simulink subsystem "PvtSubSys_PLAN_ALC"  (R2020b)
settings: Solver=VariableStepAuto  StartTime=0.0  StopTime=10.0  RelTol=1e-3
undefined symbols (not defined in the file or in its folder): P_Global_WheelBase_m, P_Global_WheelTrack_m, P_PLAN_ALC_DPCConfirmTimeHMI, P_PLAN_ALC_DPCExtraMultiFrameConfirmCntDrv, P_PLAN_ALC_DPCExtraMultiFrameConfirmCntNoh, P_PLAN_ALC_DPCExtraMultiFrameConfirmCntOverTk, P_PLAN_ALC_DPCthresholdLcDrvLv1, P_PLAN_ALC_DPCthresholdLcDrvLv2, P_PLAN_ALC_DPCthresholdLcDrvLv3, P_PLAN_ALC_DynamicDPCthreshold, P_PLAN_ALC_FWheelPreTime, P_PLAN_ALC_LcCancelDPCThreshold, P_PLAN_ALC_LcCancelLaneChangeReqDspTimeCnt, P_PLAN_ALC_LcCancelRoadWidthOffset, P_PLAN_ALC_LcCancelRoadWidthOffsetForDPC, P_PLAN_ALC_LcCurvatureInhibitionValueBrkPoints, P_PLAN_ALC_LcCurvatureInhibitionValueTable, P_PLAN_ALC_LcDelayCntSetNoh, P_PLAN_ALC_LcDelayCntSetOverTk, P_PLAN_ALC_LCDeltaTmeGap, P_PLAN_ALC_LcDrv_DyDiffThreshold, P_PLAN_ALC_LcDrvHMILineValidFtime, P_PLAN_ALC_LcEnterLane_factor, P_PLAN_ALC_LcFinishDyDiffBrkPoint, P_PLAN_ALC_LcFinishDyDiffRwFactorForAP, P_PLAN_ALC_LcFinishDyDiffRwFactorForHMI, P_PLAN_ALC_LcFinishDyDiffTableValue, P_PLAN_ALC_LciDrvExistDefaultDisp, P_PLAN_ALC_LciOverTkDeltaSpdLv1, P_PLAN_ALC_LciOverTkDeltaSpdLv2, P_PLAN_ALC_LciOverTkDeltaSpdLv3, P_PLAN_ALC_LcOverTkDPCthreshold, P_PLAN_ALC_LcOverTkRearVehTTClimit, P_PLAN_ALC_NOHLcSwt, P_PLAN_ALC_NOHTurnSts, P_PLAN_ALC_OverTkCutOutDyRWFactor, P_PLAN_ALC_OveTkrSupDist, P_PLAN_ALC_PreCurvatureFactor, P_PLAN_ALC_PreCurvaturePreTime, P_PLAN_ALC_TurnLmpType, P_PLAN_ALC_vMinPreLC_Drv, P_PLAN_ALC_vMinPreLC_Noh, P_PLAN_ALC_vMinPreLC_OverTk, P_PLAN_LcCancelTestEnable, PLAN_ALC_DangerObjIndex, PLAN_ALC_LcCancelReason, PLAN_ALC_LcDecsLe, PLAN_ALC_LcDecsRi, PLAN_ALC_LcFeReason, PLAN_ALC_LcReason, PLAN_ALC_sts, PLAN_ALC_stsReason, PLAN_ALC_TurnLightReq
libraries: simulink x198, TrueDurationTime x21, RisingEdgeTimer x2, JumpDetectionUint x1
(part 3 of 4)

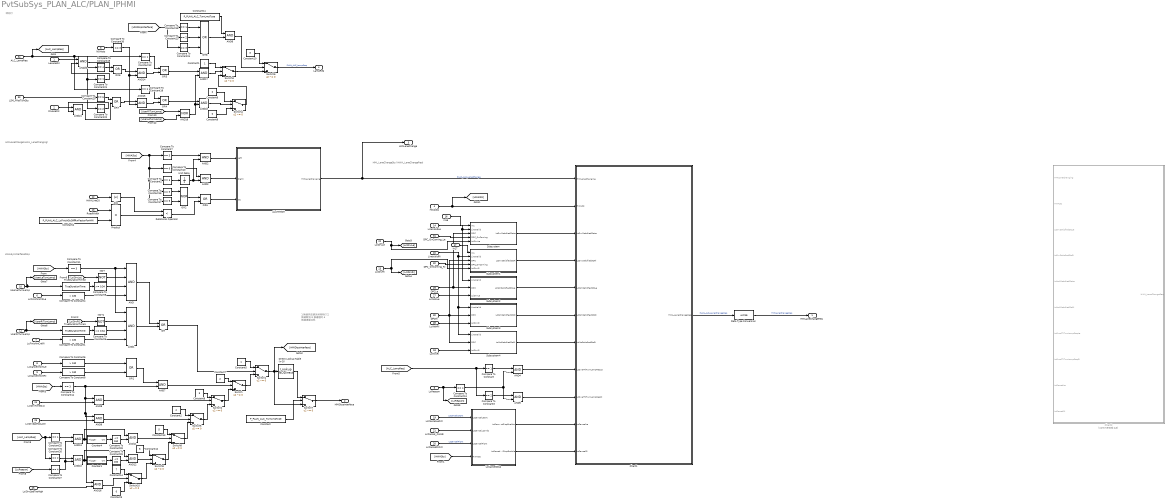
== system PvtSubSys_PLAN_ALC/PLAN_IPHMI ==
  note: 1 换道完成请关闭转向灯
      | 2 换道取消
      | 3 换道超时
      | 4 换道速度过低
  note: 转向灯
  note: HMILaneChange(HWA_LaneChanging)
  note: HMI_LaneChangeSts (HWA_LaneChangeReq)
  note: HWASysInterfaceDisp
  LeLaneOK : Inport
  RiLaneOK : Inport  Port=2
  NOHsts : Inport  Port=3
  HWASts : Inport  Port=4
  LcReason : Inport  Port=5
  LcFinishInCntLe : Inport  Port=6
  LcFinishInCntRi : Inport  Port=7
  LcCancelInCntLe : Inport  Port=8
  LcCancelInCntRi : Inport  Port=9
  UserLeTurnLamp : Inport  Port=10
  UserRiTurnLamp : Inport  Port=11
  HWALineC0 : Inport  Port=12
  RoadWidth : Inport  Port=13
  LineValidLe : Inport  Port=14
  LineValidRi : Inport  Port=15
  In16 : Inport  Port=16
  In17 : Inport  Port=17
  LcMrcRi : Inport  Port=18
  LcCancelLeCnt : Inport  Port=19
  LcCancelRiCnt : Inport  Port=20
  LcCancel_Conds : Inport  Port=21
  LciDrvLe : Inport  Port=22
  LciDrvRi : Inport  Port=23
  LciDrvTimeOut : Inport  Port=24
  LciDrvSpdTooLoW : Inport  Port=25
  LciDrvSpdTooHigh : Inport  Port=26
  LciNohLe : Inport  Port=27
  LciNohRi : Inport  Port=28
  DPCLe : Inport  Port=29
  DPCRi : Inport  Port=30
  DPC_OnComing_Le : Inport  Port=31
  DPC_OnComing_Ri : Inport  Port=32
  LSM_PilotTurnSts : Inport  Port=33
  ALC_LampReq : Inport  Port=34
  ALCHMISM : Stateflow chart  TreatAsAtomicUnit=on
  AND : Logic  Inputs=4  AllPortsSameDT=off  OutDataTypeStr=boolean
  AND1 : Logic  Inputs=4  AllPortsSameDT=off  OutDataTypeStr=boolean
  AND{2..3,6..18,20..21} (17 alike) : Logic  AllPortsSameDT=off  OutDataTypeStr=boolean
  AND19 : Logic  Operator=NOR  AllPortsSameDT=off  OutDataTypeStr=boolean
  AND4 : Logic  IconShape=distinctive  AllPortsSameDT=off  OutDataTypeStr=boolean
  AND5 : Logic  IconShape=distinctive  AllPortsSameDT=off  OutDataTypeStr=boolean
  Abs : Abs
  Chart1 : Stateflow chart  TreatAsAtomicUnit=on
  Chart2 : Stateflow chart  Commented=on  TreatAsAtomicUnit=on
  Compare To Constant{,12,15,21,25} (5 alike) : simulink/Logic and Bit Operations/Compare To Constant  relop===  const=1  OutDataTypeStr=boolean
  Compare To Constant{1,4,6,8} (4 alike) : simulink/Logic and Bit Operations/Compare To Constant  relop=>  const=130  OutDataTypeStr=boolean
  Compare To Constant10 : simulink/Logic and Bit Operations/Compare To Constant  relop===  const=6  OutDataTypeStr=boolean
  Compare To Constant{2,11,14,24,30} (5 alike) : simulink/Logic and Bit Operations/Compare To Constant  relop===  const=3  OutDataTypeStr=boolean
  Compare To Constant13 : simulink/Logic and Bit Operations/Compare To Constant  relop===  const=4  OutDataTypeStr=boolean
  Compare To Constant16 : simulink/Logic and Bit Operations/Compare To Constant  relop===  const=5  OutDataTypeStr=boolean
  Compare To Constant17 : simulink/Logic and Bit Operations/Compare To Constant  relop===  const=6  OutDataTypeStr=boolean
  Compare To Constant{3,18,22..23,26} (5 alike) : simulink/Logic and Bit Operations/Compare To Constant  relop===  const=2  OutDataTypeStr=boolean
  Compare To Constant19 : simulink/Logic and Bit Operations/Compare To Constant  relop===  const=4  OutDataTypeStr=boolean
  Compare To Constant20 : simulink/Logic and Bit Operations/Compare To Constant  relop===  const=5  OutDataTypeStr=boolean
  Compare To Constant27 : simulink/Logic and Bit Operations/Compare To Constant  relop===  const=4  OutDataTypeStr=boolean
  Compare To Constant28 : simulink/Logic and Bit Operations/Compare To Constant  relop=<=  const=150  OutDataTypeStr=boolean
  Compare To Constant29 : simulink/Logic and Bit Operations/Compare To Constant  relop=<=  const=150  OutDataTypeStr=boolean
  Compare To Constant5 : simulink/Logic and Bit Operations/Compare To Constant  relop=>=  const=0.34  OutDataTypeStr=boolean
  Compare To Constant7 : simulink/Logic and Bit Operations/Compare To Constant  relop===  const=5  OutDataTypeStr=boolean
  Compare To Constant9 : simulink/Logic and Bit Operations/Compare To Constant  relop=>=  const=0.34  OutDataTypeStr=boolean
  Constant : Constant  Value=P_PLAN_ALC_TurnLmpType
  Constant1 : Constant  OutDataTypeStr=uint8
  Constant10 : Constant  Value=3  OutDataTypeStr=uint8
  Constant11 : Constant  Value=P_PLAN_ALC_TurnLmpType
  Constant12 : Constant  Value=6  OutDataTypeStr=Inherit: Inherit via back propagation
  Constant13 : Constant  Value=5  OutDataTypeStr=Inherit: Inherit via back propagation
  Constant14 : Constant  Value=7  OutDataTypeStr=Inherit: Inherit via back propagation
  Constant2 : Constant  Value=4  OutDataTypeStr=Inherit: Inherit via back propagation
  Constant3 : Constant  Value=0  OutDataTypeStr=Inherit: Inherit via back propagation
  Constant4 : Constant  Value=P_PLAN_ALC_LcFinishDyDiffRwFactorForHMI
  Constant5 : Constant  OutDataTypeStr=Inherit: Inherit via back propagation
  Constant6 : Constant  Value=2  OutDataTypeStr=uint8
  Constant7 : Constant  Value=2  OutDataTypeStr=Inherit: Inherit via back propagation
  Constant8 : Constant  Value=3  OutDataTypeStr=Inherit: Inherit via back propagation
  Constant9 : Constant  Value=0  OutDataTypeStr=uint8
  Counter1 : Subsystem
  Counter4 : Subsystem
  Data Type Conversion : DataTypeConversion  OutDataTypeStr=uint16
  Direct Lookup Table (n-D) : LookupNDDirect  NumberOfTableDimensions=1  Table=[0 0 2 3 4 ]  DiagnosticForOutOfRangeInput=Error  TableDataTypeStr=uint8
  LcCancelDisp : Subsystem
  NOT : Logic  Operator=NOT  IconShape=distinctive  AllPortsSameDT=off  OutDataTypeStr=boolean
  NOT1 : Logic  Operator=NOT  IconShape=distinctive  AllPortsSameDT=off  OutDataTypeStr=boolean
  OR{,1,3..7} (7 alike) : Logic  Operator=OR  AllPortsSameDT=off  OutDataTypeStr=boolean
  OR2 : Logic  Operator=NOR  AllPortsSameDT=off  OutDataTypeStr=boolean
  OR8 : Logic  Operator=OR  Inputs=3  AllPortsSameDT=off  OutDataTypeStr=boolean
  Product : Product
  Relational Operator : RelationalOperator  Operator=<  OutDataTypeStr=boolean  RndMeth=Simplest
  Subsystem : Subsystem
  Subsystem1 : Subsystem
  Subsystem2 : Subsystem
  Subsystem3 : Subsystem
  Subsystem4 : Subsystem
  Switch{,1..10} (11 alike) : Switch  Criteria=u2 ~= 0
  TrueDurationTime1 : TrueDurationTime/TrueDurationTime  TCycle=0.02
  TrueDurationTime2 : TrueDurationTime/TrueDurationTime  TCycle=0.02
  Unit Delay : UnitDelay  SampleTime=-1  HasFrameUpgradeWarning=on
  HMILaneChangeReq : Outport
  HMIDispInterface : Outport  Port=2
  HMILaneChange : Outport  Port=3
  LampReq : Outport  Port=4
  wires:
  In17/1 -> Subsystem1/1(In1)
  In16/1 -> Subsystem/1(In1)
  [UserLeTurnLamp] -> AND19/2
  [UserRiTurnLamp] -> AND19/1
  AND18/1 -> Switch4/2
  AND19/1 -> AND18/2, AND17/2
  AND17/1 -> Switch3/2
  AND16/1 -> Switch10/2
  LciDrvSpdTooHigh/1 -> AND16/2
  Constant14/1 -> Switch10/1
  Switch10/1 -> Switch9/3
  Compare To Constant30/1 -> AND15/2, AND14/2
  AND13/1 -> Counter4/1(Trigger), AND11/1
  Constant13/1 -> Switch8/1
  AND12/1 -> Switch9/2
  AND11/1 -> Switch8/2
  [LcReason] -> Compare To Constant27/1
  Constant12/1 -> Switch9/1
  Compare To Constant26/1 -> AND10/1
  Compare To Constant27/1 -> AND10/2, AND13/2
  [ALC_LampReq] -> Compare To Constant25/1, Compare To Constant26/1
  Compare To Constant25/1 -> AND13/1
  Constant3/1 -> Switch10/3
  Counter1/1(Cnt) -> Compare To Constant29/1
  Compare To Constant29/1 -> AND12/2
  Counter4/1(Cnt) -> Compare To Constant28/1
  Compare To Constant28/1 -> AND11/2
  AND10/1 -> Counter1/1(Trigger), AND12/1
  Switch9/1 -> Switch8/3
  Switch8/1 -> Switch5/3
  Constant1/1 -> Switch3/1
  Constant9/1 -> Switch4/3
  LSM_PilotTurnSts/1 -> Compare To Constant22/1, Compare To Constant20/1, Compare To Constant19/1, Compare To Constant21/1
  Switch6/1 -> LampReq/1  "PLAN_ALC_LampReq"
  Compare To Constant21/1 -> AND20/2
  OR6/1 -> AND14/1
  Constant6/1 -> Switch4/1
  Compare To Constant12/1 -> OR3/1
  Switch4/1 -> Switch3/3
  Compare To Constant22/1 -> AND21/2
  ALC_LampReq/1 -> Compare To Constant12/1, Compare To Constant18/1, [ALC_LampReq]
  Compare To Constant20/1 -> OR7/1
  Compare To Constant19/1 -> OR6/1
  Compare To Constant18/1 -> OR4/1
  OR3/1 -> AND17/1
  AND15/1 -> OR4/2
  OR4/1 -> AND18/1
  ALCHMISM/1(HMILaneChanging) -> Chart1/1(HMILaneChanging), HMILaneChange/1  "PLAN_ALC_LaneChange"
  OR2/1 -> OR5/1
  Relational Operator/1 -> OR5/2
  Product/1 -> Relational Operator/2
  Abs/1 -> Relational Operator/1
  Compare To Constant13/1 -> AND4/2, AND5/2
  LcReason/1 -> Compare To Constant13/1, [LcReason]
  Compare To Constant/1 -> AND4/1
  Compare To Constant3/1 -> AND5/1
  AND5/1 -> Chart1/9(LcOverTkTurnLampReqRi)
  AND4/1 -> Chart1/8(LcOverTkTurnLampReqLe)
  [ALC_LampReq] -> Compare To Constant/1, Compare To Constant3/1
  [HWASts] -> LcCancelDisp/4(HWASts)
  LcCancelDisp/2(LcCancelRiDispEnable) -> Chart1/11(LcCancelRi)
  LcCancelDisp/1(LcCancelLeDispEnable) -> Chart1/10(LcCancelLe)
  LcCancelRiCnt/1 -> LcCancelDisp/3(LcCancelRiCnt)  "LcCancelRiCnt"
  LcCancel_Conds/1 -> LcCancelDisp/2(LcCancel_Conds)
  LcCancelLeCnt/1 -> LcCancelDisp/1(LcCancelLeCnt)  "LcCancelLeCnt"
  LciDrvSpdTooLoW/1 -> AND9/2
  LciDrvTimeOut/1 -> AND8/2
  OR1/1 -> AND7/1
  Compare To Constant14/1 -> AND8/1, AND9/1, AND16/1, AND7/2
  [HWASts] -> Compare To Constant14/1
  Compare To Constant11/1 -> AND/1, AND1/1
  [HWASts] -> Compare To Constant11/1
  [LciDrvRi] -> NOT1/1
  [LciDrvLe] -> NOT/1
  LciNohRi/1 -> Subsystem3/3(LciDrvRi)
  LciNohLe/1 -> Subsystem2/3(LciDrvLe)
  LineValidRi/1 -> Subsystem1/2(LineValid), Subsystem4/1(LineValid), Subsystem3/1(LineValid)
  LineValidLe/1 -> Subsystem/2(LineValid), Subsystem2/1(LineValid)
  DPC_OnComing_Ri/1 -> Subsystem1/4(DPC_OnComing)
  DPC_OnComing_Le/1 -> Subsystem/4(DPC_OnComing)
  DPCRi/1 -> Subsystem4/2(DPC), Subsystem3/2(DPC), Subsystem1/3(DPC)
  DPCLe/1 -> Subsystem2/2(DPC), Subsystem/3(DPC)
  LciDrvRi/1 -> Subsystem1/5(LciDrvRi), [LciDrvRi]
  LciDrvLe/1 -> Subsystem/5(LciDrvLe), [LciDrvLe]
  Subsystem3/1(LcNohSatisfiedStsRi) -> Chart1/6(LcNohSatisfiedStsRi)
  Subsystem2/1(LcNohSatisfiedStsLe) -> Chart1/5(LcNohSatisfiedStsLe)
  Unit Delay/1 -> AND2/2, AND3/2
  Constant4/1 -> Product/2
  RoadWidth/1 -> Product/1
  AND3/1 -> ALCHMISM/2(Right)
  AND2/1 -> ALCHMISM/1(Left)
  OR5/1 -> ALCHMISM/3(CC)
  [HWASts] -> Compare To Constant7/1, Compare To Constant10/1, Compare To Constant17/1, Compare To Constant16/1, Compare To Constant2/1
  Compare To Constant2/1 -> Unit Delay/1
  HWALineC0/1 -> Abs/1
  Compare To Constant7/1 -> AND2/1
  Compare To Constant10/1 -> AND3/1
  Compare To Constant8/1 -> OR1/2
  Compare To Constant6/1 -> OR1/1
  UserRiTurnLamp/1 -> [UserRiTurnLamp], TrueDurationTime1/1
  Compare To Constant5/1 -> AND1/3
  TrueDurationTime1/1 -> Compare To Constant5/1
  Compare To Constant9/1 -> AND/3
  UserLeTurnLamp/1 -> [UserLeTurnLamp], TrueDurationTime2/1
  TrueDurationTime2/1 -> Compare To Constant9/1
  NOT1/1 -> AND1/2
  Compare To Constant1/1 -> AND1/4
  Compare To Constant4/1 -> AND/4
  NOT/1 -> AND/2
  LcCancelInCntRi/1 -> Compare To Constant8/1
  LcCancelInCntLe/1 -> Compare To Constant6/1
  LcFinishInCntLe/1 -> Compare To Constant4/1
  LcFinishInCntRi/1 -> Compare To Constant1/1
  AND/1 -> OR/1
  AND1/1 -> OR/2
  Subsystem1/1(LcDrvSatisfiedStsRi) -> Chart1/4(LcDrvSatisfiedStsRi)
  Switch5/1 -> Switch2/3
  AND9/1 -> Switch5/2
  Constant2/1 -> Switch5/1
  Subsystem/1(LcDrvSatisfiedStsLe) -> Chart1/3(LcDrvSatisfiedStsLe)
  Switch1/1 -> Direct Lookup Table (n-D)/1, [HMIDispInterface], Switch7/3
  Chart1/1(HWA_LaneChangeReq) -> Data Type Conversion/1  "PLAN_ALC_LaneChangeReq"
  Switch/1 -> Switch1/3
  OR/1 -> Switch1/2
  Constant8/1 -> Switch2/1
  Constant5/1 -> Switch1/1
  Constant7/1 -> Switch/1
  AND8/1 -> Switch2/2
  Switch2/1 -> Switch/3
  AND7/1 -> Switch/2
  Data Type Conversion/1 -> HMILaneChangeReq/1  "HMILaneChangeReq"
  HWASts/1 -> Chart1/2(HWAsts), [HWASts]
  Compare To Constant16/1 -> OR2/1
  Compare To Constant17/1 -> OR2/2
  LcMrcRi/1 -> Subsystem4/3(LciDrvRi)
  Subsystem4/1(LcMrcSatisfiedStsRi) -> Chart1/7(LcMrcSatisfiedStsRi)
  [HMIDispInterface] -> Compare To Constant24/1, Compare To Constant23/1, Compare To Constant15/1
  Compare To Constant24/1 -> OR8/3
  Compare To Constant23/1 -> OR8/2
  Compare To Constant15/1 -> OR8/1
  AND6/1 -> Switch6/2
  Switch3/1 -> Switch6/3
  Constant10/1 -> Switch6/1
  Direct Lookup Table (n-D)/1 -> Switch7/1
  Constant/1 -> Switch7/2
  Switch7/1 -> HMIDispInterface/1
  Constant11/1 -> AND6/1
  OR8/1 -> AND6/2
  AND14/1 -> OR3/2
  NOHsts/1 -> Compare To Constant30/1
  OR7/1 -> AND15/1
  LeLaneOK/1 -> AND20/1
  RiLaneOK/1 -> AND21/1
  AND20/1 -> OR6/2
  AND21/1 -> OR7/2

== system PvtSubSys_PLAN_ALC/WorkCond ==
  HWAsts : Inport
  Compare To Constant : simulink/Logic and Bit Operations/Compare To Constant  relop===  const=3  OutDataTypeStr=boolean
  Compare To Constant1 : simulink/Logic and Bit Operations/Compare To Constant  relop===  const=5  OutDataTypeStr=boolean
  Compare To Constant2 : simulink/Logic and Bit Operations/Compare To Constant  relop===  const=6  OutDataTypeStr=boolean
  OR2 : Logic  Operator=OR  Inputs=3  AllPortsSameDT=off  OutDataTypeStr=boolean
  Active : Outport
  wires:
  HWAsts/1 -> Compare To Constant2/1, Compare To Constant/1, Compare To Constant1/1
  Compare To Constant1/1 -> OR2/2
  Compare To Constant/1 -> OR2/1
  Compare To Constant2/1 -> OR2/3
  OR2/1 -> Active/1

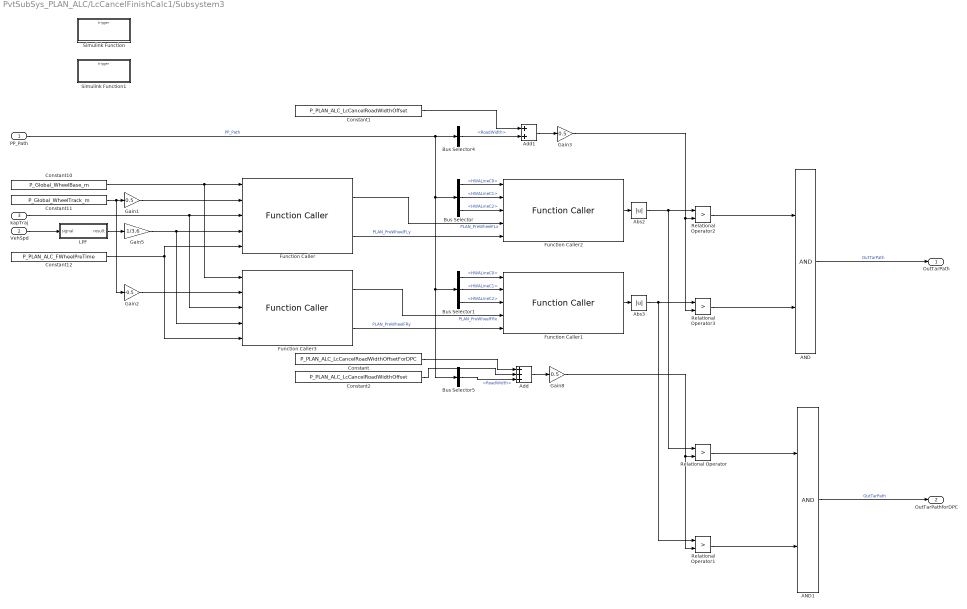
== system PvtSubSys_PLAN_ALC/LcCancelFinishCalc1/Subsystem3 ==
  PP_Path : Inport
  VehSpd : Inport  Port=2
  kapTraj : Inport  Port=3
  AND : Logic  AllPortsSameDT=off  OutDataTypeStr=boolean
  AND1 : Logic  AllPortsSameDT=off  OutDataTypeStr=boolean
  Abs2 : Abs
  Abs3 : Abs
  Add : Sum  Inputs=+++
  Add1 : Sum
  Bus Selector : BusSelector  OutputSignals=HWALineC0,HWALineC1,HWALineC2
  Bus Selector1 : BusSelector  OutputSignals=HWALineC0,HWALineC1,HWALineC2
  Bus Selector4 : BusSelector  OutputSignals=RoadWidth
  Bus Selector5 : BusSelector  OutputSignals=RoadWidth
  Constant : Constant  Value=P_PLAN_ALC_LcCancelRoadWidthOffsetForDPC
  Constant1 : Constant  Value=P_PLAN_ALC_LcCancelRoadWidthOffset
  Constant10 : Constant  Value=P_Global_WheelBase_m
  Constant11 : Constant  Value=P_Global_WheelTrack_m
  Constant12 : Constant  Value=P_PLAN_ALC_FWheelPreTime
  Constant2 : Constant  Value=P_PLAN_ALC_LcCancelRoadWidthOffset
  Function Caller : FunctionCaller  FunctionPrototype=[mPrePointX,mPrePointY] = Subsystem3.PointPre(mPointX,mPointY,kapTraj,mpsTrajSpd,sPreTime)  InputArgumentSpecifications=<Enter example>  OutputArgumentSpecifications=<Enter example>
  Function Caller1 : FunctionCaller  FunctionPrototype=PointFrenetD = Subsystem3.FrenetCS(LaneC0,LaneC1,LaneC2,PointX,PointY)  InputArgumentSpecifications=<Enter example>  OutputArgumentSpecifications=<Enter example>
  Function Caller2 : FunctionCaller  FunctionPrototype=PointFrenetD = Subsystem3.FrenetCS(LaneC0,LaneC1,LaneC2,PointX,PointY)  InputArgumentSpecifications=<Enter example>  OutputArgumentSpecifications=<Enter example>
  Function Caller3 : FunctionCaller  FunctionPrototype=[mPrePointX,mPrePointY] = Subsystem3.PointPre(mPointX,mPointY,kapTraj,mpsTrajSpd,sPreTime)  InputArgumentSpecifications=<Enter example>  OutputArgumentSpecifications=<Enter example>
  Gain1 : Gain  Gain=0.5  OutDataTypeStr=Inherit: Same as input
  Gain2 : Gain  Gain=-0.5  OutDataTypeStr=Inherit: Same as input
  Gain3 : Gain  Gain=0.5  OutDataTypeStr=Inherit: Same as input
  Gain5 : Gain  Gain=1/3.6  OutDataTypeStr=Inherit: Same as input
  Gain8 : Gain  Gain=0.5  OutDataTypeStr=Inherit: Same as input
  LPF : Subsystem
  Relational Operator{,1..3} (4 alike) : RelationalOperator  Operator=>  OutDataTypeStr=boolean  RndMeth=Simplest
  Simulink Function : Subsystem  TreatAsAtomicUnit=on
  Simulink Function1 : Subsystem  TreatAsAtomicUnit=on
  OutTarPath : Outport  OutDataTypeStr=boolean
  OutTarPathforDPC : Outport  Port=2  OutDataTypeStr=boolean
  wires:
  Constant2/1 -> Add/2
  Constant1/1 -> Add1/1
  Function Caller/1 -> Function Caller2/4  "PLAN_PreWheelFLx"
  Function Caller3/1 -> Function Caller1/4  "PLAN_PreWheelFRx"
  Function Caller3/2 -> Function Caller1/5  "PLAN_PreWheelFRy"
  Function Caller/2 -> Function Caller2/5  "PLAN_PreWheelFLy"
  AND/1 -> OutTarPath/1  "OutTarPath"
  VehSpd/1 -> LPF/1(signal)
  LPF/1(result) -> Gain5/1
  Constant11/1 -> Gain2/1, Gain1/1
  Constant10/1 -> Function Caller3/1, Function Caller/1
  Gain1/1 -> Function Caller/2
  Gain2/1 -> Function Caller3/2
  Constant12/1 -> Function Caller/5, Function Caller3/5
  Bus Selector/1 -> Function Caller2/1  "<HWALineC0>"
  Bus Selector/2 -> Function Caller2/2  "<HWALineC1>"
  Bus Selector/3 -> Function Caller2/3  "<HWALineC2>"
  Bus Selector1/3 -> Function Caller1/3  "<HWALineC2>"
  Bus Selector1/2 -> Function Caller1/2  "<HWALineC1>"
  Bus Selector1/1 -> Function Caller1/1  "<HWALineC0>"
  Add1/1 -> Gain3/1
  kapTraj/1 -> Function Caller3/3, Function Caller/3
  Add/1 -> Gain8/1
  AND1/1 -> OutTarPathforDPC/1  "OutTarPath"
  PP_Path/1 -> Bus Selector5/1, Bus Selector1/1, Bus Selector/1, Bus Selector4/1  "PP_Path"
  Relational Operator/1 -> AND1/1
  Relational Operator1/1 -> AND1/2
  Gain5/1 -> Function Caller3/4, Function Caller/4
  Bus Selector5/1 -> Add/3  "<RoadWidth>"
  Constant/1 -> Add/1
  Abs2/1 -> Relational Operator2/1, Relational Operator/1
  Abs3/1 -> Relational Operator1/1, Relational Operator3/1
  Gain8/1 -> Relational Operator1/2, Relational Operator/2
  Gain3/1 -> Relational Operator2/2, Relational Operator3/2
  Relational Operator3/1 -> AND/2
  Relational Operator2/1 -> AND/1
  Function Caller2/1 -> Abs2/1
  Function Caller1/1 -> Abs3/1
  Bus Selector4/1 -> Add1/2  "<RoadWidth>"

== system PvtSubSys_PLAN_ALC/LcDrv/Counter1 ==
  Trigger : Inport
  Constant3 : Constant  OutDataTypeStr=uint16
  Constant4 : Constant  Value=0  OutDataTypeStr=uint16
  Saturation1 : Saturate  UpperLimit=65000  LowerLimit=0
  Sum : Sum  Inputs=++|
  Switch : Switch  Criteria=u2 ~= 0
  Switch1 : Switch  Criteria=u2 ~= 0
  Unit Delay : UnitDelay  SampleTime=-1  HasFrameUpgradeWarning=on
  Cnt : Outport
  wires:
  Saturation1/1 -> Unit Delay/1, Cnt/1
  Sum/1 -> Switch1/1
  Trigger/1 -> Switch1/2, Switch/2
  Unit Delay/1 -> Sum/1
  Switch/1 -> Sum/2
  Switch1/1 -> Saturation1/1
  Constant3/1 -> Switch/1
  Constant4/1 -> Switch1/3, Switch/3

== system PvtSubSys_PLAN_ALC/LcDrv/Counter2 ==
  Trigger : Inport
  Constant3 : Constant  OutDataTypeStr=uint16
  Constant4 : Constant  Value=0  OutDataTypeStr=uint16
  Saturation1 : Saturate  UpperLimit=65000  LowerLimit=0
  Sum : Sum  Inputs=++|
  Switch : Switch  Criteria=u2 ~= 0
  Switch1 : Switch  Criteria=u2 ~= 0
  Unit Delay : UnitDelay  SampleTime=-1  HasFrameUpgradeWarning=on
  Cnt : Outport
  wires:
  Constant4/1 -> Switch/3, Switch1/3
  Constant3/1 -> Switch/1
  Switch1/1 -> Saturation1/1
  Switch/1 -> Sum/2
  Unit Delay/1 -> Sum/1
  Trigger/1 -> Switch/2, Switch1/2
  Sum/1 -> Switch1/1
  Saturation1/1 -> Cnt/1, Unit Delay/1

== system PvtSubSys_PLAN_ALC/LcDrv/Counter3 ==
  Trigger : Inport
  Constant3 : Constant  OutDataTypeStr=uint16
  Constant4 : Constant  Value=0  OutDataTypeStr=uint16
  Saturation1 : Saturate  UpperLimit=65000  LowerLimit=0
  Sum : Sum  Inputs=++|
  Switch : Switch  Criteria=u2 ~= 0
  Switch1 : Switch  Criteria=u2 ~= 0
  Unit Delay : UnitDelay  SampleTime=-1  HasFrameUpgradeWarning=on
  Cnt : Outport
  wires:
  Constant4/1 -> Switch/3, Switch1/3
  Constant3/1 -> Switch/1
  Switch1/1 -> Saturation1/1
  Switch/1 -> Sum/2
  Unit Delay/1 -> Sum/1
  Trigger/1 -> Switch/2, Switch1/2
  Sum/1 -> Switch1/1
  Saturation1/1 -> Cnt/1, Unit Delay/1

== system PvtSubSys_PLAN_ALC/LcDrv/Counter4 ==
  Trigger : Inport
  Constant3 : Constant  OutDataTypeStr=uint16
  Constant4 : Constant  Value=0  OutDataTypeStr=uint16
  Saturation1 : Saturate  UpperLimit=65000  LowerLimit=0
  Sum : Sum  Inputs=++|
  Switch : Switch  Criteria=u2 ~= 0
  Switch1 : Switch  Criteria=u2 ~= 0
  Unit Delay : UnitDelay  SampleTime=-1  HasFrameUpgradeWarning=on
  Cnt : Outport
  wires:
  Saturation1/1 -> Unit Delay/1, Cnt/1
  Sum/1 -> Switch1/1
  Trigger/1 -> Switch1/2, Switch/2
  Unit Delay/1 -> Sum/1
  Switch/1 -> Sum/2
  Switch1/1 -> Saturation1/1
  Constant3/1 -> Switch/1
  Constant4/1 -> Switch1/3, Switch/3

== system PvtSubSys_PLAN_ALC/LcDrv/Counter5 ==
  Trigger : Inport
  Constant3 : Constant  OutDataTypeStr=uint16
  Constant4 : Constant  Value=0  OutDataTypeStr=uint16
  Saturation1 : Saturate  UpperLimit=65000  LowerLimit=0
  Sum : Sum  Inputs=++|
  Switch : Switch  Criteria=u2 ~= 0
  Switch1 : Switch  Criteria=u2 ~= 0
  Unit Delay : UnitDelay  SampleTime=-1  HasFrameUpgradeWarning=on
  Cnt : Outport
  wires:
  Saturation1/1 -> Unit Delay/1, Cnt/1
  Sum/1 -> Switch1/1
  Trigger/1 -> Switch1/2, Switch/2
  Unit Delay/1 -> Sum/1
  Switch/1 -> Sum/2
  Switch1/1 -> Saturation1/1
  Constant3/1 -> Switch/1
  Constant4/1 -> Switch1/3, Switch/3

== system PvtSubSys_PLAN_ALC/LcDrv/Counter6 ==
  Trigger : Inport
  Constant3 : Constant  OutDataTypeStr=uint16
  Constant4 : Constant  Value=0  OutDataTypeStr=uint16
  Saturation1 : Saturate  UpperLimit=65000  LowerLimit=0
  Sum : Sum  Inputs=++|
  Switch : Switch  Criteria=u2 ~= 0
  Switch1 : Switch  Criteria=u2 ~= 0
  Unit Delay : UnitDelay  SampleTime=-1  HasFrameUpgradeWarning=on
  Cnt : Outport
  wires:
  Constant4/1 -> Switch/3, Switch1/3
  Constant3/1 -> Switch/1
  Switch1/1 -> Saturation1/1
  Switch/1 -> Sum/2
  Unit Delay/1 -> Sum/1
  Trigger/1 -> Switch/2, Switch1/2
  Sum/1 -> Switch1/1
  Saturation1/1 -> Cnt/1, Unit Delay/1

== system PvtSubSys_PLAN_ALC/LcDrv/Subsystem ==
  User_ALC_Swt : Inport
  Compare To Constant : simulink/Logic and Bit Operations/Compare To Constant  relop===  const=1  OutDataTypeStr=boolean
  Compare To Constant1 : simulink/Logic and Bit Operations/Compare To Constant  relop===  const=2  OutDataTypeStr=boolean
  Compare To Constant2 : simulink/Logic and Bit Operations/Compare To Constant  relop===  const=3  OutDataTypeStr=boolean
  LCDeltaTmeGap : Constant  Value=P_PLAN_ALC_LCDeltaTmeGap
  P0DeltaSpd_kph3 : Constant  Value=P_PLAN_ALC_DPCthresholdLcDrvLv1
  P0DeltaSpd_kph4 : Constant  Value=P_PLAN_ALC_DPCthresholdLcDrvLv2
  P0DeltaSpd_kph5 : Constant  Value=P_PLAN_ALC_DPCthresholdLcDrvLv3
  Switch1 : Switch  Criteria=u2 ~= 0
  Switch2 : Switch  Criteria=u2 ~= 0
  Switch9 : Switch  Criteria=u2 ~= 0
  Terminator1 : Terminator
  DPCthreshold : Outport
  wires:
  LCDeltaTmeGap/1 -> Terminator1/1
  Compare To Constant2/1 -> Switch9/2
  Compare To Constant1/1 -> Switch2/2
  Compare To Constant/1 -> Switch1/2
  User_ALC_Swt/1 -> Compare To Constant/1, Compare To Constant1/1, Compare To Constant2/1
  Switch2/1 -> Switch1/3
  Switch9/1 -> Switch2/3
  Switch1/1 -> DPCthreshold/1
  P0DeltaSpd_kph3/1 -> Switch1/1
  P0DeltaSpd_kph4/1 -> Switch2/1, Switch9/3
  P0DeltaSpd_kph5/1 -> Switch9/1

== system PvtSubSys_PLAN_ALC/LcMrc/Counter6 ==
  Trigger : Inport
  Constant3 : Constant  OutDataTypeStr=uint16
  Constant4 : Constant  Value=0  OutDataTypeStr=uint16
  Saturation1 : Saturate  UpperLimit=65000  LowerLimit=0
  Sum : Sum  Inputs=++|
  Switch : Switch  Criteria=u2 ~= 0
  Switch1 : Switch  Criteria=u2 ~= 0
  Unit Delay : UnitDelay  SampleTime=-1  HasFrameUpgradeWarning=on
  Cnt : Outport
  wires:
  Constant4/1 -> Switch/3, Switch1/3
  Constant3/1 -> Switch/1
  Switch1/1 -> Saturation1/1
  Switch/1 -> Sum/2
  Unit Delay/1 -> Sum/1
  Trigger/1 -> Switch/2, Switch1/2
  Sum/1 -> Switch1/1
  Saturation1/1 -> Cnt/1, Unit Delay/1

== system PvtSubSys_PLAN_ALC/LcNoh/Counter1 ==
  Trigger : Inport
  Constant3 : Constant  OutDataTypeStr=uint16
  Constant4 : Constant  Value=0  OutDataTypeStr=uint16
  Saturation1 : Saturate  UpperLimit=65000  LowerLimit=0
  Sum : Sum  Inputs=++|
  Switch : Switch  Criteria=u2 ~= 0
  Switch1 : Switch  Criteria=u2 ~= 0
  Unit Delay : UnitDelay  SampleTime=-1  HasFrameUpgradeWarning=on
  Cnt : Outport
  wires:
  Saturation1/1 -> Unit Delay/1, Cnt/1
  Sum/1 -> Switch1/1
  Trigger/1 -> Switch1/2, Switch/2
  Unit Delay/1 -> Sum/1
  Switch/1 -> Sum/2
  Switch1/1 -> Saturation1/1
  Constant3/1 -> Switch/1
  Constant4/1 -> Switch1/3, Switch/3

== system PvtSubSys_PLAN_ALC/LcNoh/Counter6 ==
  Trigger : Inport
  Constant3 : Constant  OutDataTypeStr=uint16
  Constant4 : Constant  Value=0  OutDataTypeStr=uint16
  Saturation1 : Saturate  UpperLimit=65000  LowerLimit=0
  Sum : Sum  Inputs=++|
  Switch : Switch  Criteria=u2 ~= 0
  Switch1 : Switch  Criteria=u2 ~= 0
  Unit Delay : UnitDelay  SampleTime=-1  HasFrameUpgradeWarning=on
  Cnt : Outport
  wires:
  Constant4/1 -> Switch/3, Switch1/3
  Constant3/1 -> Switch/1
  Switch1/1 -> Saturation1/1
  Switch/1 -> Sum/2
  Unit Delay/1 -> Sum/1
  Trigger/1 -> Switch/2, Switch1/2
  Sum/1 -> Switch1/1
  Saturation1/1 -> Cnt/1, Unit Delay/1

== system PvtSubSys_PLAN_ALC/LcOverTk/Counter1 ==
  Trigger : Inport
  Constant3 : Constant  OutDataTypeStr=uint16
  Constant4 : Constant  Value=0  OutDataTypeStr=uint16
  Saturation1 : Saturate  UpperLimit=65000  LowerLimit=0
  Sum : Sum  Inputs=++|
  Switch : Switch  Criteria=u2 ~= 0
  Switch1 : Switch  Criteria=u2 ~= 0
  Unit Delay : UnitDelay  SampleTime=-1  HasFrameUpgradeWarning=on
  Cnt : Outport
  wires:
  Saturation1/1 -> Unit Delay/1, Cnt/1
  Sum/1 -> Switch1/1
  Trigger/1 -> Switch1/2, Switch/2
  Unit Delay/1 -> Sum/1
  Switch/1 -> Sum/2
  Switch1/1 -> Saturation1/1
  Constant3/1 -> Switch/1
  Constant4/1 -> Switch1/3, Switch/3

== system PvtSubSys_PLAN_ALC/LcOverTk/Counter2 ==
  Trigger : Inport
  Constant3 : Constant  OutDataTypeStr=uint16
  Constant4 : Constant  Value=0  OutDataTypeStr=uint16
  Saturation1 : Saturate  UpperLimit=65000  LowerLimit=0
  Sum : Sum  Inputs=++|
  Switch : Switch  Criteria=u2 ~= 0
  Switch1 : Switch  Criteria=u2 ~= 0
  Unit Delay : UnitDelay  SampleTime=-1  HasFrameUpgradeWarning=on
  Cnt : Outport
  wires:
  Constant4/1 -> Switch/3, Switch1/3
  Constant3/1 -> Switch/1
  Switch1/1 -> Saturation1/1
  Switch/1 -> Sum/2
  Unit Delay/1 -> Sum/1
  Trigger/1 -> Switch/2, Switch1/2
  Sum/1 -> Switch1/1
  Saturation1/1 -> Cnt/1, Unit Delay/1

== system PvtSubSys_PLAN_ALC/LcOverTk/DrvCancelSup ==
  DrvTurnLamp : Inport
  CancelLe : Inport  Port=2
  CancelRi : Inport  Port=3
  LcReason : Inport  Port=4
  V_ego : Inport  Port=5
  LCKsts : Inport  Port=6
  User_DrvOverride : Inport  Port=7
  ALC_sts : Inport  Port=8
  AND : Logic  Inputs=3  AllPortsSameDT=off  OutDataTypeStr=boolean
  AND1 : Logic  IconShape=distinctive  AllPortsSameDT=off  OutDataTypeStr=boolean
  Chart : Stateflow chart  TreatAsAtomicUnit=on
  Compare To Constant1 : simulink/Logic and Bit Operations/Compare To Constant  relop===  const=2  OutDataTypeStr=boolean
  Compare To Constant2 : simulink/Logic and Bit Operations/Compare To Constant  relop===  const=4  OutDataTypeStr=boolean
  Compare To Constant3 : simulink/Logic and Bit Operations/Compare To Constant  relop=>  const=P_PLAN_ALC_OveTkrSupDist  OutDataTypeStr=boolean
  Compare To Constant4 : simulink/Logic and Bit Operations/Compare To Constant  relop===  const=3  OutDataTypeStr=boolean
  JumpDetectionUint2 : JumpDetectionUint/JumpDetectionUint  StartValue=3  FinishValue=2
  OR : Logic  Operator=OR  IconShape=distinctive  AllPortsSameDT=off  OutDataTypeStr=boolean
  OR1 : Logic  Operator=OR  IconShape=distinctive  AllPortsSameDT=off  OutDataTypeStr=boolean
  OR2 : Logic  Operator=OR  AllPortsSameDT=off  OutDataTypeStr=boolean
  Terminator : Terminator
  Unit Delay : UnitDelay  SampleTime=-1  HasFrameUpgradeWarning=on
  OveTkrSup_DrvCancel : Outport
  wires:
  OR2/1 -> AND/2
  CancelRi/1 -> OR2/1
  CancelLe/1 -> OR2/2
  OR1/1 -> Chart/1(Trigger)
  AND1/1 -> OR1/2
  AND/1 -> OR1/1
  OR/1 -> AND1/2
  User_DrvOverride/1 -> AND1/1
  Compare To Constant4/1 -> OR/2
  Compare To Constant1/1 -> OR/1
  ALC_sts/1 -> Compare To Constant1/1, Compare To Constant4/1
  Chart/1(Sts) -> OveTkrSup_DrvCancel/1  "OveTkrDrvCancelSup"
  LcReason/1 -> Compare To Constant2/1
  V_ego/1 -> Chart/2(V_ego)
  Compare To Constant3/1 -> Chart/3(Clear)
  DrvTurnLamp/1 -> AND/1
  Chart/2(dis) -> Unit Delay/1  "PLAN_ALC_OveTkrSupDist"
  Unit Delay/1 -> Compare To Constant3/1
  Compare To Constant2/1 -> AND/3
  LCKsts/1 -> JumpDetectionUint2/1
  JumpDetectionUint2/1 -> Terminator/1

== system PvtSubSys_PLAN_ALC/LcOverTk/Subsystem ==
  User_ALC_Swt : Inport
  Compare To Constant : simulink/Logic and Bit Operations/Compare To Constant  relop===  const=1  OutDataTypeStr=boolean
  Compare To Constant1 : simulink/Logic and Bit Operations/Compare To Constant  relop===  const=2  OutDataTypeStr=boolean
  Compare To Constant2 : simulink/Logic and Bit Operations/Compare To Constant  relop===  const=3  OutDataTypeStr=boolean
  LCDeltaTmeGap : Constant  Value=P_PLAN_ALC_LCDeltaTmeGap
  P0DeltaSpd_kph : Constant  Value=P_PLAN_ALC_LciOverTkDeltaSpdLv1
  P0DeltaSpd_kph1 : Constant  Value=P_PLAN_ALC_LciOverTkDeltaSpdLv2
  P0DeltaSpd_kph2 : Constant  Value=P_PLAN_ALC_LciOverTkDeltaSpdLv3
  P0DeltaSpd_kph3 : Constant  Value=0.1
  P0DeltaSpd_kph4 : Constant  Value=0.05
  P0DeltaSpd_kph5 : Constant  Value=0
  Switch{1..5,9} (6 alike) : Switch  Criteria=u2 ~= 0
  Terminator1 : Terminator
  DeltaSpd : Outport
  DPCthreshold : Outport  Port=2
  wires:
  P0DeltaSpd_kph5/1 -> Switch9/1
  P0DeltaSpd_kph4/1 -> Switch9/3, Switch2/1
  P0DeltaSpd_kph3/1 -> Switch1/1
  Switch1/1 -> DPCthreshold/1
  Switch9/1 -> Switch2/3
  Switch2/1 -> Switch1/3
  User_ALC_Swt/1 -> Compare To Constant2/1, Compare To Constant1/1, Compare To Constant/1
  Switch4/1 -> Switch3/3
  Switch5/1 -> Switch4/3
  Compare To Constant/1 -> Switch3/2, Switch1/2
  Compare To Constant1/1 -> Switch4/2, Switch2/2
  Compare To Constant2/1 -> Switch5/2, Switch9/2
  Switch3/1 -> DeltaSpd/1
  P0DeltaSpd_kph/1 -> Switch3/1
  P0DeltaSpd_kph1/1 -> Switch4/1, Switch5/3
  P0DeltaSpd_kph2/1 -> Switch5/1
  LCDeltaTmeGap/1 -> Terminator1/1

== system PvtSubSys_PLAN_ALC/LcOverTk/Subsystem4 ==
  P0ID : Inport
  P0Dx : Inport  Port=2
  P0Dy : Inport  Port=3
  P0Vy : Inport  Port=4
  LaneWidth : Inport  Port=5
  HWALineValid : Inport  Port=6
  " HWALineC3" : Inport  Port=7
  HWALineC2 : Inport  Port=8
  HWALineC1 : Inport  Port=9
  HWALineC0 : Inport  Port=10
  HWALineRange : Inport  Port=11
  Add : Sum
  Compare To Constant1 : simulink/Logic and Bit Operations/Compare To Constant  relop=>  const=3  OutDataTypeStr=boolean
  Compare To Zero : simulink/Logic and Bit Operations/Compare To Zero  relop=~=  OutDataTypeStr=boolean
  Constant : Constant  Value=1.5
  Constant1 : Constant  Value=P_PLAN_ALC_OverTkCutOutDyRWFactor
  Constant70 : Constant  Value=3  OutDataTypeStr=single
  Gain : Gain  Gain=-1
  MATLAB Function : MATLAB Function  TreatAsAtomicUnit=on
  OR2 : Logic  Operator=OR  AllPortsSameDT=off  OutDataTypeStr=boolean
  OR3 : Logic  Operator=OR  AllPortsSameDT=off  OutDataTypeStr=boolean
  Product : Product
  Product1 : Product
  Product2 : Product
  Relational Operator : RelationalOperator  Operator=>  OutDataTypeStr=boolean  RndMeth=Simplest
  Relational Operator1 : RelationalOperator  Operator=<  OutDataTypeStr=boolean  RndMeth=Simplest
  Relational Operator2 : RelationalOperator  Operator=>  OutDataTypeStr=boolean  RndMeth=Simplest
  Relational Operator3 : RelationalOperator  Operator=<  OutDataTypeStr=boolean  RndMeth=Simplest
  SLPDyCalc : MATLAB Function  TreatAsAtomicUnit=on
  Switch2 : Switch  Criteria=u2 ~= 0
  Unit Delay : UnitDelay  SampleTime=-1  HasFrameUpgradeWarning=on
  Unit Delay1 : UnitDelay  SampleTime=-1  HasFrameUpgradeWarning=on
  LcOverTkSup_LeP0CutOut : Outport
  LcOverTkSup_RiP0CutOut : Outport  Port=2
  wires:
  Product2/1 -> Gain/1
  Constant1/1 -> Product2/1, Product1/1
  P0Dy/1 -> SLPDyCalc/2(ObjDy)
  P0Dx/1 -> SLPDyCalc/1(ObjDx)
  " HWALineC3"/1 -> SLPDyCalc/4(LineC3)
  HWALineC2/1 -> SLPDyCalc/5(LineC2)
  HWALineC1/1 -> SLPDyCalc/6(LineC1)
  HWALineC0/1 -> SLPDyCalc/7(LineC0)
  HWALineRange/1 -> SLPDyCalc/8(LineRange)
  HWALineValid/1 -> SLPDyCalc/3(LineValid)
  Gain/1 -> Relational Operator3/2, Relational Operator1/2  "Ri"
  Product1/1 -> Relational Operator/2, Relational Operator2/2  "Le"
  Compare To Constant1/1 -> Switch2/2
  Constant70/1 -> Switch2/3
  LaneWidth/1 -> Compare To Constant1/1, Switch2/1
  Relational Operator1/1 -> OR3/2
  Relational Operator/1 -> OR2/2
  Switch2/1 -> Product1/2, Product2/2
  Relational Operator3/1 -> OR3/1  "RightCutOut"
  Relational Operator2/1 -> OR2/1  "LeftCutOut"
  Constant/1 -> Product/2
  Unit Delay1/1 -> MATLAB Function/4(resultK1)
  MATLAB Function/1(result) -> Product/1, Unit Delay1/1
  Add/1 -> Relational Operator3/1, Relational Operator2/1  "PLAN_ALC_PreP0Dy"
  Product/1 -> Add/2
  SLPDyCalc/1(dDyDiffRelLine) -> Relational Operator/1, Relational Operator1/1, Add/1
  P0Vy/1 -> MATLAB Function/3(signal)
  OR2/1 -> LcOverTkSup_LeP0CutOut/1
  OR3/1 -> LcOverTkSup_RiP0CutOut/1
  P0ID/1 -> Compare To Zero/1
  Compare To Zero/1 -> MATLAB Function/1(Trigger), Unit Delay/1
  Unit Delay/1 -> MATLAB Function/2(TriggerK1)

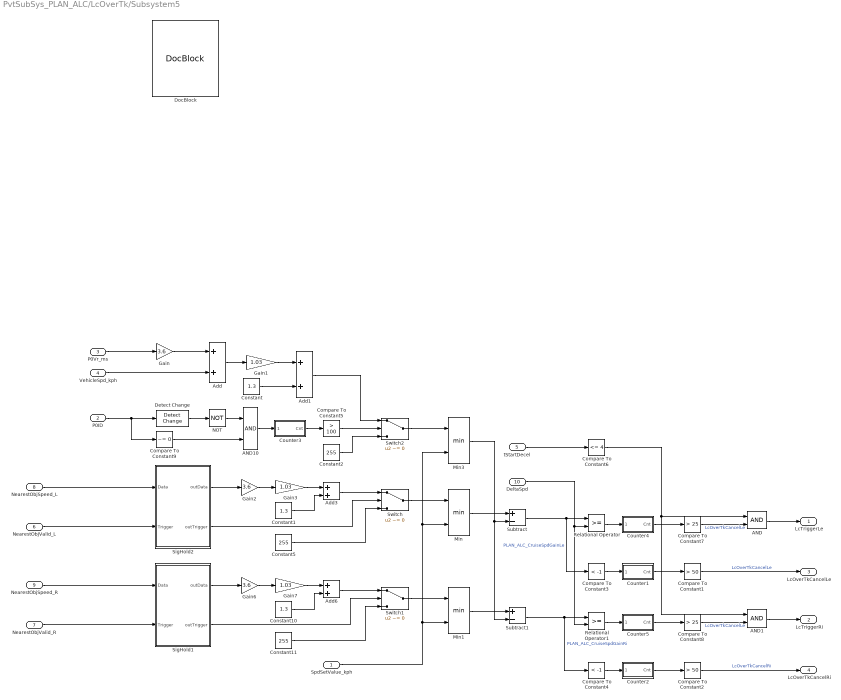
== system PvtSubSys_PLAN_ALC/LcOverTk/Subsystem5 ==
  SpdSetValue_kph : Inport
  P0ID : Inport  Port=2
  P0Vr_ms : Inport  Port=3
  VehicleSpd_kph : Inport  Port=4
  tStartDecel : Inport  Port=5
  NearestObjValid_L : Inport  Port=6
  NearestObjValid_R : Inport  Port=7
  NearestObjSpeed_L : Inport  Port=8
  NearestObjSpeed_R : Inport  Port=9
  DeltaSpd : Inport  Port=10
  AND : Logic  AllPortsSameDT=off  OutDataTypeStr=boolean
  AND1 : Logic  AllPortsSameDT=off  OutDataTypeStr=boolean
  AND10 : Logic  AllPortsSameDT=off  OutDataTypeStr=boolean
  Add{,1,3,6} (4 alike) : Sum
  Compare To Constant1 : simulink/Logic and Bit Operations/Compare To Constant  relop=>  const=50  OutDataTypeStr=boolean
  Compare To Constant2 : simulink/Logic and Bit Operations/Compare To Constant  relop=>  const=50  OutDataTypeStr=boolean
  Compare To Constant3 : simulink/Logic and Bit Operations/Compare To Constant  relop=<  const=-1  OutDataTypeStr=boolean
  Compare To Constant4 : simulink/Logic and Bit Operations/Compare To Constant  relop=<  const=-1  OutDataTypeStr=boolean
  Compare To Constant5 : simulink/Logic and Bit Operations/Compare To Constant  relop=>  const=100  OutDataTypeStr=boolean
  Compare To Constant6 : simulink/Logic and Bit Operations/Compare To Constant  relop=<=  const=4  OutDataTypeStr=boolean
  Compare To Constant7 : simulink/Logic and Bit Operations/Compare To Constant  relop=>  const=25  OutDataTypeStr=boolean
  Compare To Constant8 : simulink/Logic and Bit Operations/Compare To Constant  relop=>  const=25  OutDataTypeStr=boolean
  Compare To Constant9 : simulink/Logic and Bit Operations/Compare To Constant  relop=~=  const=0  OutDataTypeStr=boolean
  Constant : Constant  Value=1.3
  Constant1 : Constant  Value=1.3
  Constant10 : Constant  Value=1.3
  Constant11 : Constant  Value=255
  Constant2 : Constant  Value=255
  Constant5 : Constant  Value=255
  Counter1 : Subsystem
  Counter2 : Subsystem
  Counter3 : Subsystem
  Counter4 : Subsystem
  Counter5 : Subsystem
  Detect Change : simulink/Logic and Bit Operations/Detect Change  vinit=0  OutDataTypeStr=boolean
  DocBlock : simulink/Model-Wide Utilities/DocBlock  DocumentType=Text
      content=|
      | 换道触发条件
      |
      | 压速换道取消条件
  Gain : Gain  Gain=3.6
  Gain1 : Gain  Gain=1.03
  Gain2 : Gain  Gain=3.6
  Gain3 : Gain  Gain=1.03
  Gain6 : Gain  Gain=3.6
  Gain7 : Gain  Gain=1.03
  Min : MinMax  Inputs=2
  Min1 : MinMax  Inputs=2
  Min3 : MinMax  Inputs=2
  NOT : Logic  Operator=NOT  IconShape=distinctive  AllPortsSameDT=off  OutDataTypeStr=boolean
  Relational Operator : RelationalOperator  OutDataTypeStr=boolean  RndMeth=Simplest
  Relational Operator1 : RelationalOperator  OutDataTypeStr=boolean  RndMeth=Simplest
  SigHold1 : Stateflow chart  TreatAsAtomicUnit=on
  SigHold2 : Stateflow chart  TreatAsAtomicUnit=on
  Subtract : Sum  Inputs=+-
  Subtract1 : Sum  Inputs=+-
  Switch : Switch  Criteria=u2 ~= 0
  Switch1 : Switch  Criteria=u2 ~= 0
  Switch2 : Switch  Criteria=u2 ~= 0
  LcTriggerLe : Outport
  LcTriggerRi : Outport  Port=2
  LcOverTkCancelLe : Outport  Port=3
  LcOverTkCancelRi : Outport  Port=4
  wires:
  AND1/1 -> LcTriggerRi/1
  Compare To Constant6/1 -> AND/1, AND1/1
  Relational Operator/1 -> Counter4/1(Trigger)
  Relational Operator1/1 -> Counter5/1(Trigger)
  AND/1 -> LcTriggerLe/1
  Subtract1/1 -> Compare To Constant4/1, Relational Operator1/1  "PLAN_ALC_CruiseSpdGainRi"
  Subtract/1 -> Compare To Constant3/1, Relational Operator/1  "PLAN_ALC_CruiseSpdGainLe"
  VehicleSpd_kph/1 -> Add/2
  NearestObjSpeed_L/1 -> SigHold2/1(Data)
  Gain2/1 -> Gain3/1
  Gain3/1 -> Add3/1
  Constant1/1 -> Add3/2
  Add3/1 -> Switch/1
  Constant/1 -> Add1/2
  Gain1/1 -> Add1/1
  Add/1 -> Gain1/1
  Gain/1 -> Add/1
  Min/1 -> Subtract/1
  Min3/1 -> Subtract/2, Subtract1/2
  Min1/1 -> Subtract1/1
  Counter2/1(Cnt) -> Compare To Constant2/1
  Counter1/1(Cnt) -> Compare To Constant1/1
  P0Vr_ms/1 -> Gain/1
  tStartDecel/1 -> Compare To Constant6/1
  SpdSetValue_kph/1 -> Min3/2, Min/2, Min1/2
  Constant5/1 -> Switch/3
  Constant11/1 -> Switch1/3
  Add6/1 -> Switch1/1
  Constant10/1 -> Add6/2
  Gain7/1 -> Add6/1
  Gain6/1 -> Gain7/1
  NearestObjSpeed_R/1 -> SigHold1/1(Data)
  Switch/1 -> Min/1
  Switch1/1 -> Min1/1
  P0ID/1 -> Detect Change/1, Compare To Constant9/1
  Compare To Constant9/1 -> AND10/2
  Counter3/1(Cnt) -> Compare To Constant5/1
  Detect Change/1 -> NOT/1
  NOT/1 -> AND10/1
  AND10/1 -> Counter3/1(Trigger)
  SigHold2/1(outData) -> Gain2/1
  NearestObjValid_L/1 -> SigHold2/2(Trigger)
  SigHold2/2(outTrigger) -> Switch/2
  NearestObjValid_R/1 -> SigHold1/2(Trigger)
  SigHold1/2(outTrigger) -> Switch1/2
  SigHold1/1(outData) -> Gain6/1
  Add1/1 -> Switch2/1
  Compare To Constant5/1 -> Switch2/2
  Constant2/1 -> Switch2/3
  Switch2/1 -> Min3/1
  DeltaSpd/1 -> Relational Operator1/2, Relational Operator/2
  Compare To Constant3/1 -> Counter1/1(Trigger)
  Compare To Constant4/1 -> Counter2/1(Trigger)
  Compare To Constant1/1 -> LcOverTkCancelLe/1  "LcOverTkCancelLe"
  Compare To Constant2/1 -> LcOverTkCancelRi/1  "LcOverTkCancelRi"
  Counter4/1(Cnt) -> Compare To Constant7/1
  Counter5/1(Cnt) -> Compare To Constant8/1
  Compare To Constant7/1 -> AND/2  "LcOverTkCancelLe"
  Compare To Constant8/1 -> AND1/2  "LcOverTkCancelLe"

== system PvtSubSys_PLAN_ALC/PLAN_IPHMI/Counter1 ==
  Trigger : Inport
  Constant3 : Constant  OutDataTypeStr=uint16
  Constant4 : Constant  Value=0  OutDataTypeStr=uint16
  Saturation1 : Saturate  UpperLimit=65000  LowerLimit=0
  Sum : Sum  Inputs=++|
  Switch : Switch  Criteria=u2 ~= 0
  Switch1 : Switch  Criteria=u2 ~= 0
  Unit Delay : UnitDelay  SampleTime=-1  HasFrameUpgradeWarning=on
  Cnt : Outport
  wires:
  Saturation1/1 -> Unit Delay/1, Cnt/1
  Sum/1 -> Switch1/1
  Trigger/1 -> Switch1/2, Switch/2
  Unit Delay/1 -> Sum/1
  Switch/1 -> Sum/2
  Switch1/1 -> Saturation1/1
  Constant3/1 -> Switch/1
  Constant4/1 -> Switch1/3, Switch/3

== system PvtSubSys_PLAN_ALC/PLAN_IPHMI/Counter4 ==
  Trigger : Inport
  Constant3 : Constant  OutDataTypeStr=uint16
  Constant4 : Constant  Value=0  OutDataTypeStr=uint16
  Saturation1 : Saturate  UpperLimit=65000  LowerLimit=0
  Sum : Sum  Inputs=++|
  Switch : Switch  Criteria=u2 ~= 0
  Switch1 : Switch  Criteria=u2 ~= 0
  Unit Delay : UnitDelay  SampleTime=-1  HasFrameUpgradeWarning=on
  Cnt : Outport
  wires:
  Constant4/1 -> Switch/3, Switch1/3
  Constant3/1 -> Switch/1
  Switch1/1 -> Saturation1/1
  Switch/1 -> Sum/2
  Unit Delay/1 -> Sum/1
  Trigger/1 -> Switch/2, Switch1/2
  Sum/1 -> Switch1/1
  Saturation1/1 -> Cnt/1, Unit Delay/1

== system PvtSubSys_PLAN_ALC/PLAN_IPHMI/LcCancelDisp ==
  LcCancelLeCnt : Inport
  LcCancel_Conds : Inport  Port=2
  LcCancelRiCnt : Inport  Port=3
  HWASts : Inport  Port=4
  AND4 : Logic  AllPortsSameDT=off  OutDataTypeStr=boolean
  AND5 : Logic  AllPortsSameDT=off  OutDataTypeStr=boolean
  AND6 : Logic  AllPortsSameDT=off  OutDataTypeStr=boolean
  Bus Selector4 : BusSelector  OutputSignals=LcCancelsLe.PLAN_ALC_LcCancelLe_DPC,LcCancelsLe.PLAN_ALC_LcCancelLe_LineValid,LcCancelsLe.PLAN_ALC_LcCancelLe_Oncoming  OutputAsBus=on
  Bus Selector5 : BusSelector  OutputSignals=LcCancelsRi.PLAN_ALC_LcCancelRi_DPC,LcCancelsRi.PLAN_ALC_LcCancelRi_LineValid,LcCancelsRi.PLAN_ALC_LcCancelRi_Oncoming  OutputAsBus=on
  Compare To Constant13 : simulink/Logic and Bit Operations/Compare To Constant  relop===  const=0  OutDataTypeStr=boolean
  Compare To Constant3 : simulink/Logic and Bit Operations/Compare To Constant  relop=~=  const=3  OutDataTypeStr=boolean
  Constant6 : Constant  Value=P_PLAN_ALC_LcCancelLaneChangeReqDspTimeCnt
  OR2 : Logic  Operator=OR  Inputs=1  AllPortsSameDT=off  OutDataTypeStr=boolean
  OR4 : Logic  Operator=OR  Inputs=1  AllPortsSameDT=off  OutDataTypeStr=boolean
  RisingEdgeTimer1 : RisingEdgeTimer/RisingEdgeTimer  MaxCnt=P_PLAN_ALC_LcCancelLaneChangeReqDspTimeCnt
  RisingEdgeTimer2 : RisingEdgeTimer/RisingEdgeTimer  MaxCnt=P_PLAN_ALC_LcCancelLaneChangeReqDspTimeCnt
  Terminator : Terminator
  Terminator1 : Terminator
  LcCancelLeDispEnable : Outport
  LcCancelRiDispEnable : Outport  Port=2
  wires:
  LcCancelLeCnt/1 -> AND4/1
  LcCancelRiCnt/1 -> AND5/1
  RisingEdgeTimer1/1 -> LcCancelRiDispEnable/1
  Compare To Constant3/1 -> AND6/1
  AND4/1 -> RisingEdgeTimer2/1
  OR4/1 -> AND5/2
  Constant6/1 -> Compare To Constant13/1
  OR2/1 -> AND4/2
  Compare To Constant13/1 -> AND6/2
  AND5/1 -> RisingEdgeTimer1/1
  Bus Selector5/1 -> OR4/1
  RisingEdgeTimer2/1 -> LcCancelLeDispEnable/1
  LcCancel_Conds/1 -> Bus Selector5/1, Bus Selector4/1
  RisingEdgeTimer1/2 -> Terminator1/1
  AND6/1 -> RisingEdgeTimer2/2, RisingEdgeTimer1/2
  RisingEdgeTimer2/2 -> Terminator/1
  Bus Selector4/1 -> OR2/1
  HWASts/1 -> Compare To Constant3/1

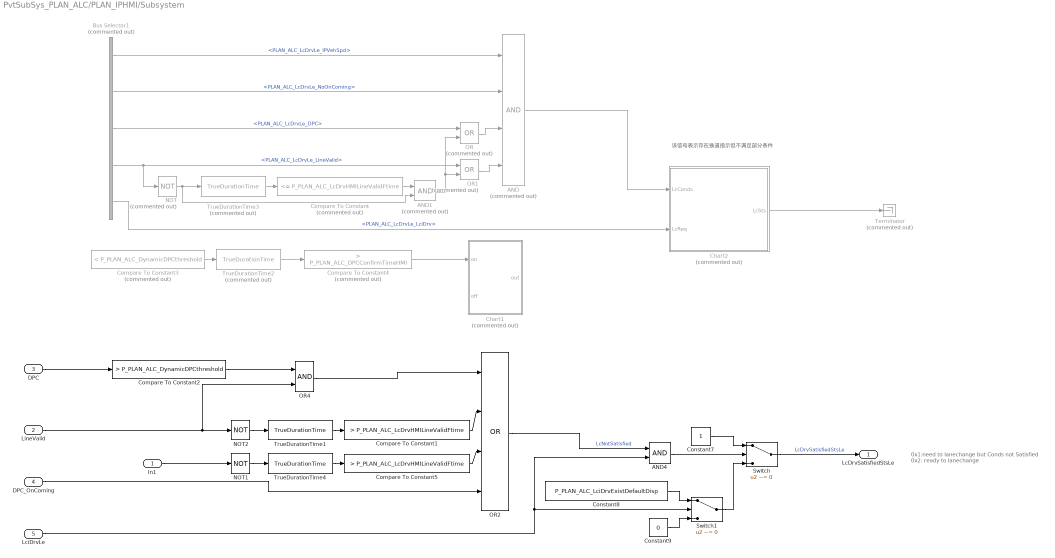
== system PvtSubSys_PLAN_ALC/PLAN_IPHMI/Subsystem ==
  note: 该信号表示存在换道指示但不满足部分条件
  note: 0x1:need to lanechange but Conds not Satisfied
      | 0x2: ready to lanechange
  In1 : Inport
  LineValid : Inport  Port=2
  DPC : Inport  Port=3
  DPC_OnComing : Inport  Port=4
  LciDrvLe : Inport  Port=5
  AND : Logic  Commented=on  Inputs=4  AllPortsSameDT=off  OutDataTypeStr=boolean
  AND1 : Logic  Commented=on  AllPortsSameDT=off  OutDataTypeStr=boolean
  AND4 : Logic  AllPortsSameDT=off  OutDataTypeStr=boolean
  Bus Selector1 : BusSelector  Commented=on  OutputSignals=PLAN_ALC_LcDrvLe_IPVehSpd,PLAN_ALC_LcDrvLe_NoOnComing,PLAN_ALC_LcDrvLe_DPC,PLAN_ALC_LcDrvLe_LineValid,PLAN_ALC_LcDrvLe_LciDrv
  Chart1 : Stateflow chart  Commented=on  TreatAsAtomicUnit=on
  Chart2 : Stateflow chart  Commented=on  TreatAsAtomicUnit=on
  Compare To Constant : simulink/Logic and Bit Operations/Compare To Constant  Commented=on  relop=<=  const=P_PLAN_ALC_LcDrvHMILineValidFtime  OutDataTypeStr=boolean
  Compare To Constant1 : simulink/Logic and Bit Operations/Compare To Constant  relop=>  const=P_PLAN_ALC_LcDrvHMILineValidFtime  OutDataTypeStr=boolean
  Compare To Constant2 : simulink/Logic and Bit Operations/Compare To Constant  relop=>  const=P_PLAN_ALC_DynamicDPCthreshold  OutDataTypeStr=boolean
  Compare To Constant3 : simulink/Logic and Bit Operations/Compare To Constant  Commented=on  relop=<  const=P_PLAN_ALC_DynamicDPCthreshold  OutDataTypeStr=boolean
  Compare To Constant4 : simulink/Logic and Bit Operations/Compare To Constant  Commented=on  relop=>  const=P_PLAN_ALC_DPCConfirmTimeHMI  OutDataTypeStr=boolean
  Compare To Constant5 : simulink/Logic and Bit Operations/Compare To Constant  relop=>  const=P_PLAN_ALC_LcDrvHMILineValidFtime  OutDataTypeStr=boolean
  Constant7 : Constant  OutDataTypeStr=uint8
  Constant8 : Constant  Value=P_PLAN_ALC_LciDrvExistDefaultDisp  OutDataTypeStr=uint8
  Constant9 : Constant  Value=0  OutDataTypeStr=uint8
  NOT : Logic  Commented=on  Operator=NOT  IconShape=distinctive  AllPortsSameDT=off  OutDataTypeStr=boolean
  NOT1 : Logic  Operator=NOT  IconShape=distinctive  AllPortsSameDT=off  OutDataTypeStr=boolean
  NOT2 : Logic  Operator=NOT  IconShape=distinctive  AllPortsSameDT=off  OutDataTypeStr=boolean
  OR : Logic  Commented=on  Operator=OR  AllPortsSameDT=off  OutDataTypeStr=boolean
  OR1 : Logic  Commented=on  Operator=OR  AllPortsSameDT=off  OutDataTypeStr=boolean
  OR2 : Logic  Operator=OR  Inputs=4  AllPortsSameDT=off  OutDataTypeStr=boolean
  OR4 : Logic  AllPortsSameDT=off  OutDataTypeStr=boolean
  Switch : Switch  Criteria=u2 ~= 0
  Switch1 : Switch  Criteria=u2 ~= 0
  Terminator : Terminator  Commented=on
  TrueDurationTime1 : TrueDurationTime/TrueDurationTime  TCycle=0.02
  TrueDurationTime2 : TrueDurationTime/TrueDurationTime  Commented=on  TCycle=0.02
  TrueDurationTime3 : TrueDurationTime/TrueDurationTime  Commented=on  TCycle=0.02
  TrueDurationTime4 : TrueDurationTime/TrueDurationTime  TCycle=0.02
  LcDrvSatisfiedStsLe : Outport
  wires:
  Compare To Constant5/1 -> OR2/3
  TrueDurationTime4/1 -> Compare To Constant5/1
  NOT1/1 -> TrueDurationTime4/1
  In1/1 -> NOT1/1
  OR4/1 -> OR2/1
  Compare To Constant4/1 -> Chart1/1(on)
  DPC/1 -> Compare To Constant2/1
  Bus Selector1/5 -> Chart2/2(LcReq)  "<PLAN_ALC_LcDrvLe_LciDrv>"
  LciDrvLe/1 -> AND4/2, Switch1/2
  Switch/1 -> LcDrvSatisfiedStsLe/1  "LcDrvSatisfiedStsLe"
  LineValid/1 -> NOT2/1, OR4/2
  Compare To Constant2/1 -> OR4/1
  Bus Selector1/2 -> AND/2  "<PLAN_ALC_LcDrvLe_NoOnComing>"
  Constant7/1 -> Switch/1
  Bus Selector1/1 -> AND/1  "<PLAN_ALC_LcDrvLe_IPVehSpd>"
  Compare To Constant1/1 -> OR2/2
  TrueDurationTime1/1 -> Compare To Constant1/1
  NOT2/1 -> TrueDurationTime1/1
  Switch1/1 -> Switch/3
  OR2/1 -> AND4/1  "LcNotSatisfied"
  Constant8/1 -> Switch1/1
  Bus Selector1/4 -> OR1/1, NOT/1  "<PLAN_ALC_LcDrvLe_LineValid>"
  AND4/1 -> Switch/2
  Bus Selector1/3 -> OR/1  "<PLAN_ALC_LcDrvLe_DPC>"
  Constant9/1 -> Switch1/3
  DPC_OnComing/1 -> OR2/4
  Compare To Constant/1 -> AND1/1
  AND/1 -> Chart2/1(LcConds)
  AND1/1 -> OR1/2, OR/2
  TrueDurationTime3/1 -> Compare To Constant/1
  NOT/1 -> TrueDurationTime3/1, AND1/2
  OR1/1 -> AND/4
  OR/1 -> AND/3
  Chart2/1(LcSts) -> Terminator/1
  Compare To Constant3/1 -> TrueDurationTime2/1
  TrueDurationTime2/1 -> Compare To Constant4/1
